simulink model "AutoBoat"  (R2018a)
settings: Solver=FixedStepAuto  StartTime=0.0  StopTime=inf  RelTol=1e-3
PreLoadFcn:
  | addpath(fullfile(fileparts(codertarget.arduinobase.internal.getBaseSpPkgRootDir), 'arduinotarget', 'arduinotargetdemos','demo_src'));
libraries: arduinolib x6
CloseFcn:
  | if (exist('GPSParser.m', 'file') ==2)
  | rmpath(fullfile(fileparts(codertarget.arduinobase.internal.getBaseSpPkgRootDir), 'arduinotarget', 'arduinotargetdemos','demo_src'));
  | end
settings Model: SimulationMode=external  ExtModeTrigDuration=2  ExtModeArchiveDirName=C:\Users\mmordeka\Desktop\2_6_morning  ExtModeAddSuffixToVar=on  Creator=The MathWorks, Inc.  LastModifiedBy=Fredrik
settings OptimizationCC: PassReuseOutputArgsThreshold=0  MaxStackSize=64
settings DebuggingCC: ParameterTunabilityLossMsg=error
settings HardwareCC: ProdBitPerInt=16  ProdBitPerPointer=16  ProdBitPerSizeT=16  ProdBitPerPtrDiffT=16  ProdLargestAtomicFloat=None  ProdWordSize=8  ProdHWDeviceType=Atmel->AVR  UseEmbeddedCoderFeatures=off  UseSimulinkCoderFeatures=off
settings SFSimCC: MATLABDynamicMemAlloc=off
settings RTWCC: SystemTargetFile=ert.tlc  HardwareBoard=Arduino Mega 2560  TLCOptions=-aInlineSetEventsForThisBaseRateFcn=TLC_FALSE -aSuppressMultiTaskScheduler=TLC_FALSE -aRateBasedStepFcn=1  TemplateMakefile=ert_default_tmf  GenerateReport=on  Toolchain=Arduino AVR  BuildConfiguration=Faster Runs  LaunchReport=on
settings CodeAppCC: ForceParamTrailComments=on  OperatorAnnotations=on  MangleLength=10  StateflowObjectComments=on  MATLABSourceComments=on
settings ERTTargetCC: ERTCustomFileBanners=off  SupportContinuousTime=on  SupportNonInlinedSFcns=on  RemoveResetFunc=off  SupportVariableSizeSignals=on  ModelStepFunctionPrototypeControlCompliant=off

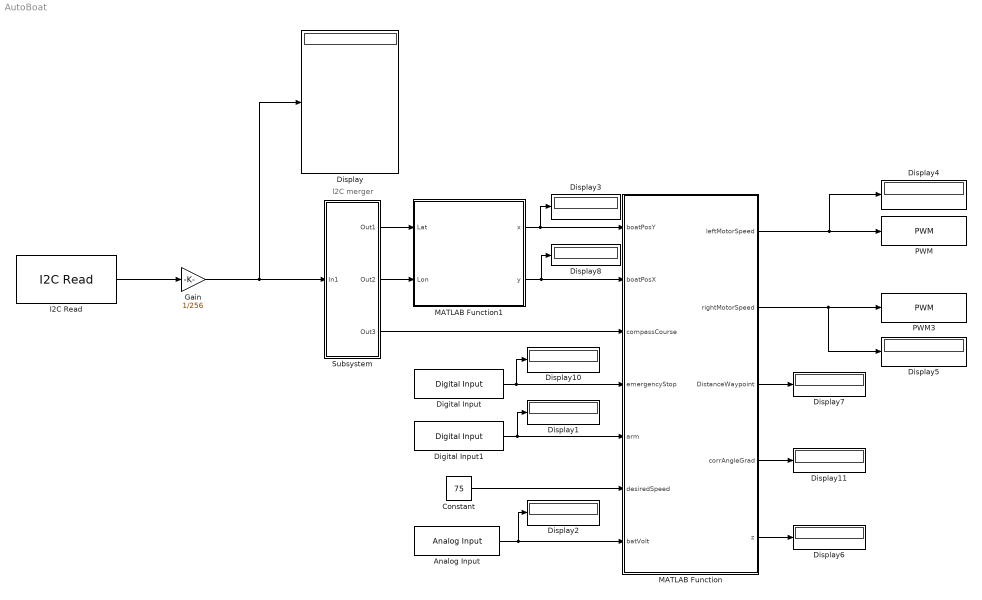
== system AutoBoat ==
  note: I2C merger
  Analog Input : arduinolib/Analog Input  pinNumber=0  ReadResultsOnly=off  ConversionTriggerSource=Software  ExternalTriggerType=uint32(0)  OutputDataType=uint16  EnableConversionCompleteNotify=off  EnableOuputStatus=off  SampleTime=1  blockPlatform=arduino
  Constant : Constant  Value=75
  Digital Input : arduinolib/Digital Input  pinNumber=30  sampleTime=0.1  blockPlatform=arduino
      settings: SourceProductName=Simulink Support Package for Arduino Hardware
  Digital Input1 : arduinolib/Digital Input  pinNumber=32  sampleTime=0.1  blockPlatform=arduino
      settings: SourceProductName=Simulink Support Package for Arduino Hardware
  Display{,1..8,10..11} (11 alike) : Display
  Gain : Gain  Gain=1/256  OutDataTypeStr=double
  I2C Read : arduinolib/I2C Read  SlaveAddress_=hex2dec( '48' )  RegisterAddressEnable=off  RegisterAddress_=hex2dec( '20' )  Datatype=uint16  ByteOrder=Big Endian  Datalength_=10  SampleTime_=0.5  blockPlatform=arduino
      settings: SourceProductName=Simulink Support Package for Arduino Hardware  SourceProductBaseCode=ARDUINO
  MATLAB Function : MATLAB Function  TreatAsAtomicUnit=on
  MATLAB Function1 : MATLAB Function  TreatAsAtomicUnit=on
  PWM : arduinolib/PWM  pinNumber=11  EnableInputFrequency=off  InitialFrequency=2000  InitialDutyCycle=0  NotificationType=None  blockPlatform=arduino
  PWM3 : arduinolib/PWM  pinNumber=12  EnableInputFrequency=off  InitialFrequency=2000  InitialDutyCycle=0  NotificationType=None  blockPlatform=arduino
  Subsystem : Subsystem
  wires:
  I2C Read/1 -> Gain/1
  MATLAB Function/3(DistanceWaypoint) -> Display7/1
  MATLAB Function/5(z) -> Display6/1
  Digital Input/1 -> Display10/1, MATLAB Function/4(emergencyStop)
  MATLAB Function/4(corrAngleGrad) -> Display11/1
  Subsystem/3(Out3) -> MATLAB Function/3(compassCourse)
  MATLAB Function/1(leftMotorSpeed) -> Display4/1, PWM/1
  MATLAB Function/2(rightMotorSpeed) -> Display5/1, PWM3/1
  Digital Input1/1 -> Display1/1, MATLAB Function/5(arm)
  Constant/1 -> MATLAB Function/6(desiredSpeed)
  Gain/1 -> Display/1, Subsystem/1(In1)
  Subsystem/1(Out1) -> MATLAB Function1/1(Lat)
  Subsystem/2(Out2) -> MATLAB Function1/2(Lon)
  MATLAB Function1/1(x) -> Display3/1, MATLAB Function/1(boatPosY)
  MATLAB Function1/2(y) -> MATLAB Function/2(boatPosX), Display8/1
  Analog Input/1 -> Display2/1, MATLAB Function/7(batVolt)

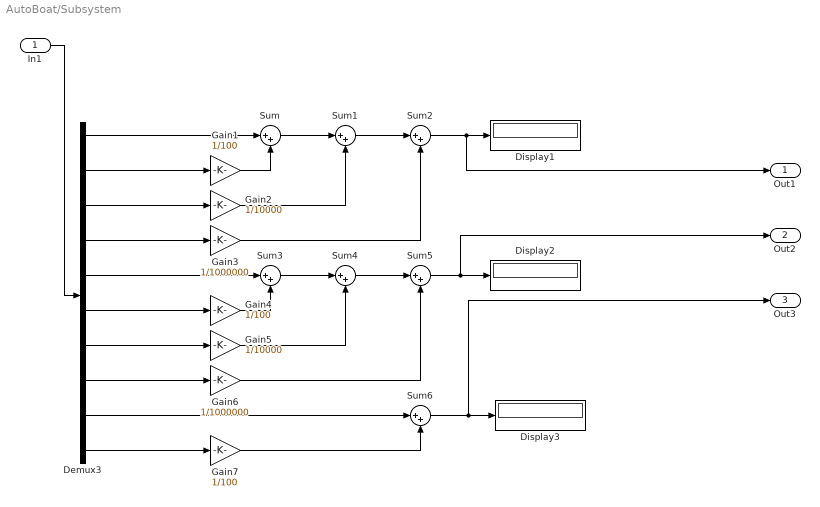
== system AutoBoat/Subsystem ==
  In1 : Inport
  Demux3 : Demux  Outputs=10
  Display1 : Display
      settings: Format=decimal (Stored Integer)
  Display2 : Display
      settings: Format=decimal (Stored Integer)
  Display3 : Display
  Gain1 : Gain  Gain=1/100
  Gain2 : Gain  Gain=1/10000
  Gain3 : Gain  Gain=1/1000000
  Gain4 : Gain  Gain=1/100
  Gain5 : Gain  Gain=1/10000
  Gain6 : Gain  Gain=1/1000000
  Gain7 : Gain  Gain=1/100
  Sum{,1..6} (7 alike) : Sum  Inputs=|++
  Out1 : Outport
  Out2 : Outport  Port=2
  Out3 : Outport  Port=3
  wires:
  Sum6/1 -> Out3/1, Display3/1
  Sum5/1 -> Out2/1, Display2/1
  Sum4/1 -> Sum5/1
  Sum3/1 -> Sum4/1
  Demux3/7 -> Gain5/1
  Sum/1 -> Sum1/1
  In1/1 -> Demux3/1
  Gain7/1 -> Sum6/2
  Demux3/1 -> Sum/1
  Gain5/1 -> Sum4/2
  Demux3/9 -> Sum6/1
  Demux3/2 -> Gain1/1
  Demux3/3 -> Gain2/1
  Sum2/1 -> Out1/1, Display1/1
  Demux3/5 -> Sum3/1
  Gain4/1 -> Sum3/2
  Gain1/1 -> Sum/2
  Demux3/4 -> Gain3/1
  Gain3/1 -> Sum2/2
  Demux3/8 -> Gain6/1
  Gain2/1 -> Sum1/2
  Gain6/1 -> Sum5/2
  Demux3/6 -> Gain4/1
  Sum1/1 -> Sum2/1
  Demux3/10 -> Gain7/1

== matlab function AutoBoat/MATLAB Function1 ==
  data: x output; Lat input; y output; Lon input
function  [x,y] = deg2utm(Lat,Lon)
% -------------------------------------------------------------------------
% [x,y,utmzone] = deg2utm(Lat,Lon)
%
% Description: Function to convert lat/lon vectors into UTM coordinates (WGS84).
% Some code has been extracted from UTM.m function by Gabriel Ruiz Martinez.
%
% Inputs:
%    Lat: Latitude vector.   Degrees.  +ddd.ddddd  WGS84
%    Lon: Longitude vector.  Degrees.  +ddd.ddddd  WGS84
%
% Outputs:
%    x, y , utmzone.   See example
%
% Example 1:
%    Lat=[40.3154333; 46.283900; 37.577833; 28.645650; 38.855550; 25.061783];
%    Lon=[-3.4857166; 7.8012333; -119.95525; -17.759533; -94.7990166; 121.640266];
%    [x,y,utmzone] = deg2utm(Lat,Lon);
%    fprintf('%7.0f ',x)
%       458731  407653  239027  230253  343898  362850
%    fprintf('%7.0f ',y)
%      4462881 5126290 4163083 3171843 4302285 2772478
%    utmzone =
%       30 T
%       32 T
%       11 S
%       28 R
%       15 S
%       51 R
%
% Example 2: If you have Lat/Lon coordinates in Degrees, Minutes and Seconds
%    LatDMS=[40 18 55.56; 46 17 2.04];
%    LonDMS=[-3 29  8.58;  7 48 4.44];
%    Lat=dms2deg(mat2dms(LatDMS)); %convert into degrees
%    Lon=dms2deg(mat2dms(LonDMS)); %convert into degrees
%    [x,y,utmzone] = deg2utm(Lat,Lon)
%
% Author: 
%   Rafael Palacios
%   Universidad Pontificia Comillas
%   Madrid, Spain
% Version: Apr/06, Jun/06, Aug/06, Aug/06
% Aug/06: fixed a problem (found by Rodolphe Dewarrat) related to southern 
%    hemisphere coordinates. 
% Aug/06: corrected m-Lint warnings
%-------------------------------------------------------------------------

% Argument checking
%
error(nargchk(2, 2, nargin));  %2 arguments required
n1=length(Lat);
n2=length(Lon);
if (n1~=n2)
   error('Lat and Lon vectors should have the same length');
end


% Memory pre-allocation
%
x=zeros(n1,1);
y=zeros(n1,1);
%utmzone(n1,:)='60 X';

% Main Loop
%
for i=1:n1
   la=Lat(i);
   lo=Lon(i);

   sa = 6378137.000000 ; sb = 6356752.314245;
         
   %e = ( ( ( sa ^ 2 ) - ( sb ^ 2 ) ) ^ 0.5 ) / sa;
   e2 = ( ( ( sa ^ 2 ) - ( sb ^ 2 ) ) ^ 0.5 ) / sb;
   e2cuadrada = e2 ^ 2;
   c = ( sa ^ 2 ) / sb;
   %alpha = ( sa - sb ) / sa;             %f
   %ablandamiento = 1 / alpha;   % 1/f

   lat = la * ( pi / 180 );
   lon = lo * ( pi / 180 );

   Huso = fix( ( lo / 6 ) + 31);
   S = ( ( Huso * 6 ) - 183 );
   deltaS = lon - ( S * ( pi / 180 ) );

   if (la<-72), Letra='C';
   elseif (la<-64), Letra='D';
   elseif (la<-56), Letra='E';
   elseif (la<-48), Letra='F';
   elseif (la<-40), Letra='G';
   elseif (la<-32), Letra='H';
   elseif (la<-24), Letra='J';
   elseif (la<-16), Letra='K';
   elseif (la<-8), Letra='L';
   elseif (la<0), Letra='M';
   elseif (la<8), Letra='N';
   elseif (la<16), Letra='P';
   elseif (la<24), Letra='Q';
   elseif (la<32), Letra='R';
   elseif (la<40), Letra='S';
   elseif (la<48), Letra='T';
   elseif (la<56), Letra='U';
   elseif (la<64), Letra='V';
   elseif (la<72), Letra='W';
   else Letra='X';
   end

   a = cos(lat) * sin(deltaS);
   epsilon = 0.5 * log( ( 1 +  a) / ( 1 - a ) );
   nu = atan( tan(lat) / cos(deltaS) ) - lat;
   v = ( c / ( ( 1 + ( e2cuadrada * ( cos(lat) ) ^ 2 ) ) ) ^ 0.5 ) * 0.9996;
   ta = ( e2cuadrada / 2 ) * epsilon ^ 2 * ( cos(lat) ) ^ 2;
   a1 = sin( 2 * lat );
   a2 = a1 * ( cos(lat) ) ^ 2;
   j2 = lat + ( a1 / 2 );
   j4 = ( ( 3 * j2 ) + a2 ) / 4;
   j6 = ( ( 5 * j4 ) + ( a2 * ( cos(lat) ) ^ 2) ) / 3;
   alfa = ( 3 / 4 ) * e2cuadrada;
   beta = ( 5 / 3 ) * alfa ^ 2;
   gama = ( 35 / 27 ) * alfa ^ 3;
   Bm = 0.9996 * c * ( lat - alfa * j2 + beta * j4 - gama * j6 );
   xx = epsilon * v * ( 1 + ( ta / 3 ) ) + 500000;
   yy = nu * v * ( 1 + ta ) + Bm;

   if (yy<0)
       yy=9999999+yy;
   end

   x(i)=xx;
   y(i)=yy;
end

== matlab function AutoBoat/MATLAB Function ==
  data: boatPosY input; boatPosX input; leftMotorSpeed output; rightMotorSpeed output; compassCourse input; emergencyStop input; arm input; desiredSpeed input; DistanceWaypoint output; corrAngleGrad output; z output; batVolt input
function [leftMotorSpeed, rightMotorSpeed, DistanceWaypoint, corrAngleGrad, z] = GuidanceNoLOS(boatPosY, boatPosX, compassCourse, emergencyStop, arm, desiredSpeed, batVolt)
%% Initial parameters
leftMotorThrustRatio = 0;
rightMotorTrhustRatio = 0;
leftMotorSpeed = 0;
rightMotorSpeed = 0;
compassAngle = 0;
minVoltBat = 12.4;
svingForsterkning = 3;

persistent i; 
if isempty(i) 
    i = 1;
end

%Declare variable used for disabling boat turning after first startup,
%to get GPS heading
persistent motorFirst;
if isempty(motorFirst)
    motorFirst = 0;
end

%Time that boat turning is disabled after first startup
startTime = 15*2;
z=0;

% Position Matrix
gps = [
475658.6 6465280.7;
475741.9 6465290.7;
475752.0 6465324.1;
475735.9 6465366.5;
475697.2 6465367.8;
475672.4 6465336.8;
475659.2 6465282.3]
pos = gps;

%initial boat position
Xc = boatPosX
Yc = boatPosY

%radius for next waypoint
Rk = 10;


if compassCourse <= 90
    compassAngle = 90*pi/180-compassCourse
elseif compassCourse > 90
    compassAngle = (360+90)*pi/180 - compassCourse
end
%% Target waypoint
    Xw = pos(i+1,2);
    Yw = pos(i+1,1);

%% Correction angle calculation
waypointAngle = atan((Yw - Yc)/(Xw-Xc))
if waypointAngle < 0
    waypointAngle = waypointAngle + 2*pi
end

%Selects correct waypointAngle
if (Yw - Yc) > 0 && pi < waypointAngle && waypointAngle < 2*pi
    waypointAngle = waypointAngle - pi

elseif (Yw - Yc) < 0 && 0 < waypointAngle && waypointAngle < pi
        waypointAngle = waypointAngle + pi
end

%Set correctionAngle and optimizes it
corrAngle = (waypointAngle - compassAngle)
if corrAngle > pi
    corrAngle = corrAngle - 2*pi
elseif corrAngle < -pi
    corrAngle = corrAngle + 2*pi
end
%% Motor Control
%Motors disable if battery voltage is below min limit
if(batVolt > (((minVoltBat*(20000/(47000+20000))/5)*1023)))
    
    %Disables boat turning for set time for first start
    if motorFirst <= startTime && emergencyStop == true
        leftMotorSpeed = desiredSpeed * 0.5 + 187.5
        rightMotorSpeed = desiredSpeed * 0.5 + 187.5
        motorFirst = motorFirst + 1;
    end
    %Relation between correction angle and thrusterspeed
    if corrAngle < 0
        leftMotorThrustRatio = 1
        rightMotorTrhustRatio = 1 + (corrAngle*svingForsterkning/(pi))
    elseif corrAngle > 0
        leftMotorThrustRatio = 1 - (corrAngle*svingForsterkning/(pi))
        rightMotorTrhustRatio = 1
    elseif corrAngle == 0
        leftMotorThrustRatio = 1
        rightMotorTrhustRatio = 1   
    end

    %prevent PWM signal to speedcontroller exceeds their limit
    if leftMotorThrustRatio < -1
        leftMotorThrustRatio = -1
    elseif leftMotorThrustRatio > 1
        leftMotorThrustRatio = 1
    end

    if rightMotorTrhustRatio < -1
        rightMotorTrhustRatio = -1
    elseif rightMotorTrhustRatio > 1
        rightMotorTrhustRatio = 1
    end

    %Set desired motorspeed
    %Emergency stop and auto ARMing of ESCs
    if emergencyStop == true && motorFirst >= startTime
        leftMotorSpeed = desiredSpeed * 0.5 * leftMotorThrustRatio + 187.5
        rightMotorSpeed = desiredSpeed * 0.5 * rightMotorTrhustRatio + 187.5
    elseif emergencyStop == false && arm ~= true
        leftMotorSpeed = 187.5;
        rightMotorSpeed = 187.5;
    elseif emergencyStop == false && arm ~= false
        leftMotorSpeed = 0;
        rightMotorSpeed = 0;
    elseif emergencyStop == true && arm ~= false
        leftMotorSpeed = 0;
        rightMotorSpeed = 0;
    end
end

%% post motorcontroll
 if (sqrt((Xw-Xc)^2+(Yw-Yc)^2) < Rk)
     i = i + 1;
 end
 % if last last waypoint is reached, motors stop
 if ((pos(i,1) == pos(end,1)) && (pos(i,2) == pos(end,2)))
    leftMotorSpeed = 0;
    rightMotorSpeed = 0;
 end
 % variables to monitor outside block is set
 DistanceWaypoint = sqrt((Xw-Xc)^2+(Yw-Yc)^2)
 z=i;
 corrAngleGrad = corrAngle*180/pi

end
